simulink model "sonar_sim"  (R2017b)
settings: Solver=FixedStepAuto  StartTime=0.0  StopTime=inf  RelTol=1e-6
InitFcn:
  | fs = 500000;
  | variance = 4096*0.1
libraries: dspsrcs4 x8
settings Model: Creator=rumma  LastModifiedBy=Michael
settings CodeAppCC: StateflowObjectComments=on
settings SimscapeCC: SimscapeNormalizeSystem=off

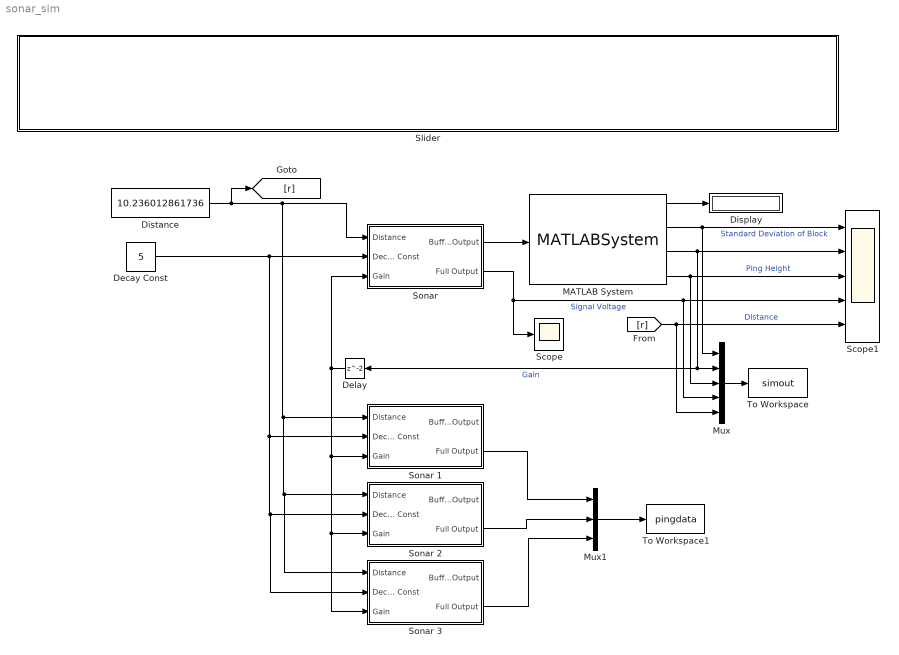
== system sonar_sim ==
  Decay Const : Constant  Value=5
  Delay : Delay
  Display : Display
      settings: Decimation=2
  Distance : Constant  Value=10.236012861736
  MATLAB System : MATLABSystem  System=GainControl  threshold_constant=3  SimulateUsing=Code generation
      mask Type: GainControl
      mask Display:
      | disp('GainControl');
      | port_label('input',1,'u');
      | port_label('output',1,'thresh');
      | port_label('output',2,'stddev');
      | port_label('output',3,'gain');
      | port_label('output',4,'pinghgt');
  Mux : Mux  Inputs=5
  Mux1 : Mux  Inputs=3
  Scope : Scope
  Scope1 : Scope  NumInputPorts=5
  Slider : Subsystem  DialogController=hmiCreateDDGDialog  IsWebBlock=on  mask(MWDashboardBlock){webBlockId=c1527e47-fbe2-4444-aee2-85079fbb3654, webBlockType=slider, ShowInLibBrowser=on, ShowInitialText=on, HMISrcModelName=sonar_sim}
      mask prompts: webBlockId "WebBlock Id"; webBlockType "WebBlock Type"; HMISrcModelName "Source Model"
      mask help: SimulinkHMI:dialogs:SliderDialogDesc
      mask Help: helpview([docroot '/mapfiles/simulink.map'], 'hmi_slider')
      mask Display:
      | if strcmp(get_param(bdroot(gcb),'BlockDiagramType'), 'library')
      |     image([(matlabroot) '/toolbox/simulink/hmi/icons/Slider.png']);
      | end
  "Sonar " : Subsystem
  Sonar 1 : Subsystem
  Sonar 2 : Subsystem
  Sonar 3 : Subsystem
  To Workspace : ToWorkspace  VariableName=simout  SaveFormat=Structure With Time  SampleTime=-1
  To Workspace1 : ToWorkspace  VariableName=pingdata  SaveFormat=Structure With Time  SampleTime=-1
  wires:
  Distance/1 -> [r], Sonar 1/1(Distance), Sonar 3/1(Distance), Sonar 2/1(Distance), "Sonar "/1(Distance)
  "Sonar "/2(Full Output) -> Mux/4, Scope1/4, Scope/1  "Signal Voltage"
  "Sonar "/1(Buffered Output) -> MATLAB System/1
  MATLAB System/2 -> Mux/1, Scope1/1  "Standard Deviation of Block"
  MATLAB System/1 -> Display/1
  MATLAB System/3 -> Delay/1, Mux/2, Scope1/2  "Gain"
  MATLAB System/4 -> Mux/3, Scope1/3  "Ping Height"
  Decay Const/1 -> Sonar 1/2(Decay Const), Sonar 3/2(Decay Const), Sonar 2/2(Decay Const), "Sonar "/2(Decay Const)
  Delay/1 -> Sonar 1/3(Gain), Sonar 3/3(Gain), Sonar 2/3(Gain), "Sonar "/3(Gain)
  [r] -> Mux/5, Scope1/5  "Distance"
  Mux/1 -> To Workspace/1
  Mux1/1 -> To Workspace1/1
  Sonar 1/2(Full Output) -> Mux1/1
  Sonar 2/2(Full Output) -> Mux1/2
  Sonar 3/2(Full Output) -> Mux1/3

== system sonar_sim/Slider ==

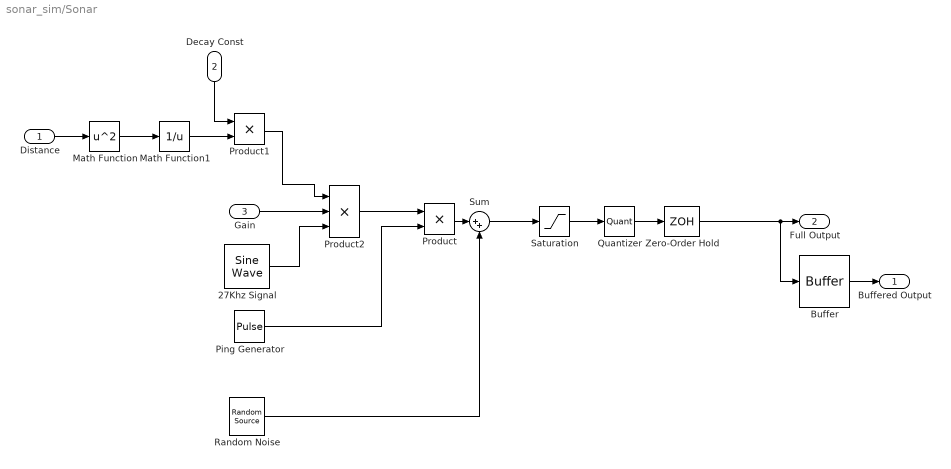
== system sonar_sim/Sonar  ==
  Distance : Inport
  Decay Const : Inport  Port=2
  Gain : Inport  Port=3
  27Khz Signal : dspsrcs4/Sine Wave  Amplitude=0.9  Frequency=27000  Phase=0  SampleMode=Discrete  OutComplex=Real  CompMethod=Trigonometric fcn  TableSize=Speed  SampleTime=1/fs  SamplesPerFrame=1  ResetState=Restart at time zero  OutputFrames=off  dataType=double  wordLen=16  udDataType=sfix(16)  fracBitsMode=Best precision  numFracBits=15  OutDataTypeStr=double  LastOutDataTypeStr=double
  Buffer : Buffer  N=256  OutputFrames=off
  Math Function : Math  Operator=square  SaturateOnIntegerOverflow=on
  Math Function1 : Math  Operator=reciprocal  SaturateOnIntegerOverflow=on
  Ping Generator : DiscretePulseGenerator  PulseType=Time based  Period=1  PulseWidth=0.4
  Product : Product  RndMeth=Convergent
  Product1 : Product
  Product2 : Product  Inputs=3
  Quantizer : Quantizer  QuantizationInterval=2/1024
  Random Noise : dspsrcs4/Random Source  SrcType=Gaussian  NormMethod=Ziggurat  CltLength=12  MinVal=0  MaxVal=1  MeanVal=1  VarVal=0.001  RepMode=Not repeatable  rawSeed=1  IsInherit=off  SampMode=Discrete  SampTime=1/fs  SampFrame=1  DataType=Double  OutComplex=Real  OutputFrames=off
  Saturation : Saturate  UpperLimit=2  LowerLimit=0
  Sum : Sum  Inputs=|++
  Zero-Order Hold : ZeroOrderHold  SampleTime=1/fs
  Buffered Output : Outport
  Full Output : Outport  Port=2
  wires:
  27Khz Signal/1 -> Product2/3
  Product1/1 -> Product2/1
  Math Function1/1 -> Product1/2
  Decay Const/1 -> Product1/1
  Math Function/1 -> Math Function1/1
  Ping Generator/1 -> Product/2
  Product/1 -> Sum/1
  Sum/1 -> Saturation/1
  Distance/1 -> Math Function/1
  Random Noise/1 -> Sum/2
  Saturation/1 -> Quantizer/1
  Quantizer/1 -> Zero-Order Hold/1
  Buffer/1 -> Buffered Output/1
  Gain/1 -> Product2/2
  Product2/1 -> Product/1
  Zero-Order Hold/1 -> Buffer/1, Full Output/1

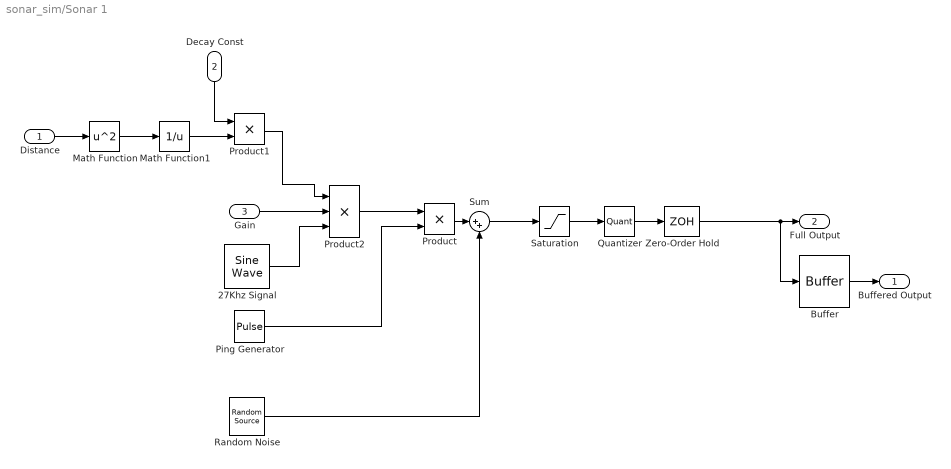
== system sonar_sim/Sonar 1 ==
  Distance : Inport
  Decay Const : Inport  Port=2
  Gain : Inport  Port=3
  27Khz Signal : dspsrcs4/Sine Wave  Amplitude=0.9*4096  Frequency=27000  Phase=0  SampleMode=Discrete  OutComplex=Real  CompMethod=Trigonometric fcn  TableSize=Speed  SampleTime=1/fs  SamplesPerFrame=1  ResetState=Restart at time zero  OutputFrames=off  dataType=double  wordLen=16  udDataType=sfix(16)  fracBitsMode=Best precision  numFracBits=15  OutDataTypeStr=double  LastOutDataTypeStr=double
  Buffer : Buffer  N=256  OutputFrames=off
  Math Function : Math  Operator=square  SaturateOnIntegerOverflow=on
  Math Function1 : Math  Operator=reciprocal  SaturateOnIntegerOverflow=on
  Ping Generator : DiscretePulseGenerator  PulseType=Time based  Period=1  PulseWidth=0.4
  Product : Product  RndMeth=Convergent
  Product1 : Product
  Product2 : Product  Inputs=3
  Quantizer : Quantizer  QuantizationInterval=1
  Random Noise : dspsrcs4/Random Source  SrcType=Gaussian  NormMethod=Ziggurat  CltLength=12  MinVal=0  MaxVal=1  MeanVal=2048  VarVal=variance  RepMode=Not repeatable  rawSeed=1  IsInherit=off  SampMode=Discrete  SampTime=1/fs  SampFrame=1  DataType=Double  OutComplex=Real  OutputFrames=off
  Saturation : Saturate  UpperLimit=4096  LowerLimit=0
  Sum : Sum  Inputs=|++
  Zero-Order Hold : ZeroOrderHold  SampleTime=1/fs
  Buffered Output : Outport
  Full Output : Outport  Port=2
  wires:
  27Khz Signal/1 -> Product2/3
  Product1/1 -> Product2/1
  Math Function1/1 -> Product1/2
  Decay Const/1 -> Product1/1
  Math Function/1 -> Math Function1/1
  Ping Generator/1 -> Product/2
  Product/1 -> Sum/1
  Sum/1 -> Saturation/1
  Distance/1 -> Math Function/1
  Random Noise/1 -> Sum/2
  Saturation/1 -> Quantizer/1
  Quantizer/1 -> Zero-Order Hold/1
  Buffer/1 -> Buffered Output/1
  Gain/1 -> Product2/2
  Product2/1 -> Product/1
  Zero-Order Hold/1 -> Buffer/1, Full Output/1

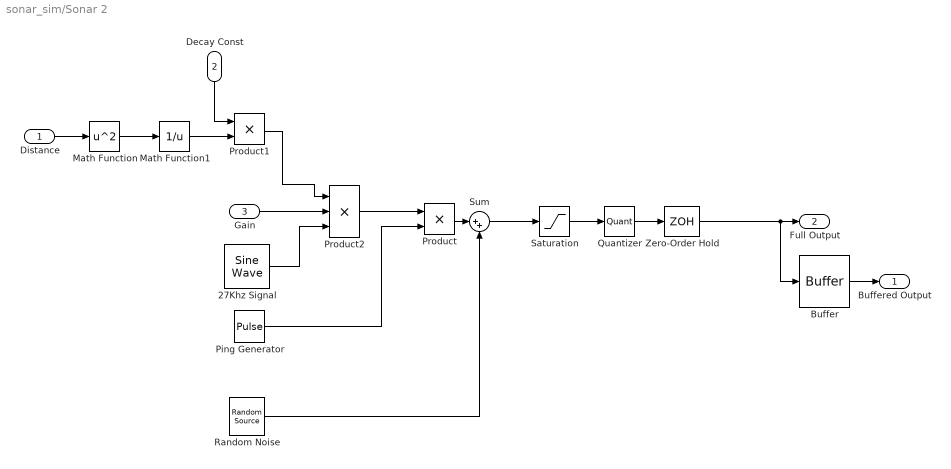
== system sonar_sim/Sonar 2 ==
  Distance : Inport
  Decay Const : Inport  Port=2
  Gain : Inport  Port=3
  27Khz Signal : dspsrcs4/Sine Wave  Amplitude=0.9*4096  Frequency=27000  Phase=0  SampleMode=Discrete  OutComplex=Real  CompMethod=Trigonometric fcn  TableSize=Speed  SampleTime=1/fs  SamplesPerFrame=1  ResetState=Restart at time zero  OutputFrames=off  dataType=double  wordLen=16  udDataType=sfix(16)  fracBitsMode=Best precision  numFracBits=15  OutDataTypeStr=double  LastOutDataTypeStr=double
  Buffer : Buffer  N=256  OutputFrames=off
  Math Function : Math  Operator=square  SaturateOnIntegerOverflow=on
  Math Function1 : Math  Operator=reciprocal  SaturateOnIntegerOverflow=on
  Ping Generator : DiscretePulseGenerator  PulseType=Time based  Period=1  PulseWidth=0.4
  Product : Product  RndMeth=Convergent
  Product1 : Product
  Product2 : Product  Inputs=3
  Quantizer : Quantizer  QuantizationInterval=1
  Random Noise : dspsrcs4/Random Source  SrcType=Gaussian  NormMethod=Ziggurat  CltLength=12  MinVal=0  MaxVal=1  MeanVal=2048  VarVal=variance  RepMode=Not repeatable  rawSeed=1  IsInherit=off  SampMode=Discrete  SampTime=1/fs  SampFrame=1  DataType=Double  OutComplex=Real  OutputFrames=off
  Saturation : Saturate  UpperLimit=4096  LowerLimit=0
  Sum : Sum  Inputs=|++
  Zero-Order Hold : ZeroOrderHold  SampleTime=1/fs
  Buffered Output : Outport
  Full Output : Outport  Port=2
  wires:
  27Khz Signal/1 -> Product2/3
  Product1/1 -> Product2/1
  Math Function1/1 -> Product1/2
  Decay Const/1 -> Product1/1
  Math Function/1 -> Math Function1/1
  Ping Generator/1 -> Product/2
  Product/1 -> Sum/1
  Sum/1 -> Saturation/1
  Distance/1 -> Math Function/1
  Random Noise/1 -> Sum/2
  Saturation/1 -> Quantizer/1
  Quantizer/1 -> Zero-Order Hold/1
  Buffer/1 -> Buffered Output/1
  Gain/1 -> Product2/2
  Product2/1 -> Product/1
  Zero-Order Hold/1 -> Buffer/1, Full Output/1

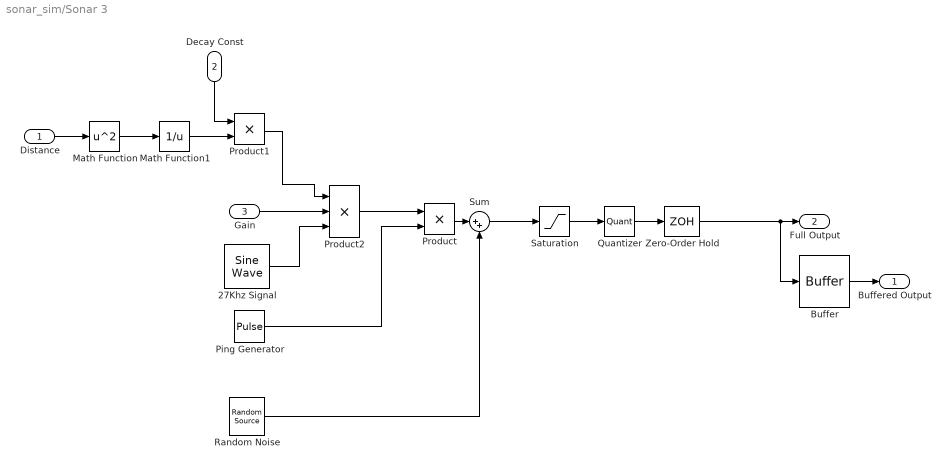
== system sonar_sim/Sonar 3 ==
  Distance : Inport
  Decay Const : Inport  Port=2
  Gain : Inport  Port=3
  27Khz Signal : dspsrcs4/Sine Wave  Amplitude=0.9*4096  Frequency=27000  Phase=0  SampleMode=Discrete  OutComplex=Real  CompMethod=Trigonometric fcn  TableSize=Speed  SampleTime=1/fs  SamplesPerFrame=1  ResetState=Restart at time zero  OutputFrames=off  dataType=double  wordLen=16  udDataType=sfix(16)  fracBitsMode=Best precision  numFracBits=15  OutDataTypeStr=double  LastOutDataTypeStr=double
  Buffer : Buffer  N=256  OutputFrames=off
  Math Function : Math  Operator=square  SaturateOnIntegerOverflow=on
  Math Function1 : Math  Operator=reciprocal  SaturateOnIntegerOverflow=on
  Ping Generator : DiscretePulseGenerator  PulseType=Time based  Period=1  PulseWidth=0.4
  Product : Product  RndMeth=Convergent
  Product1 : Product
  Product2 : Product  Inputs=3
  Quantizer : Quantizer  QuantizationInterval=1
  Random Noise : dspsrcs4/Random Source  SrcType=Gaussian  NormMethod=Ziggurat  CltLength=12  MinVal=0  MaxVal=1  MeanVal=2048  VarVal=variance  RepMode=Not repeatable  rawSeed=1  IsInherit=off  SampMode=Discrete  SampTime=1/fs  SampFrame=1  DataType=Double  OutComplex=Real  OutputFrames=off
  Saturation : Saturate  UpperLimit=4096  LowerLimit=0
  Sum : Sum  Inputs=|++
  Zero-Order Hold : ZeroOrderHold  SampleTime=1/fs
  Buffered Output : Outport
  Full Output : Outport  Port=2
  wires:
  27Khz Signal/1 -> Product2/3
  Product1/1 -> Product2/1
  Math Function1/1 -> Product1/2
  Decay Const/1 -> Product1/1
  Math Function/1 -> Math Function1/1
  Ping Generator/1 -> Product/2
  Product/1 -> Sum/1
  Sum/1 -> Saturation/1
  Distance/1 -> Math Function/1
  Random Noise/1 -> Sum/2
  Saturation/1 -> Quantizer/1
  Quantizer/1 -> Zero-Order Hold/1
  Buffer/1 -> Buffered Output/1
  Gain/1 -> Product2/2
  Product2/1 -> Product/1
  Zero-Order Hold/1 -> Buffer/1, Full Output/1
